simulink model "SiDynoReferenceApplication"  (R2020a)
settings: Solver=ode23tb  StartTime=0.0  StopTime=15000  RelTol=1e-3  EnableMultiTasking=on
model workspace (MAT data in the model file):
  DynOperatingPts : timeseries (value not decoded)
  MaxTurboSpd = 232000
  SteadyEngSpdCmdPts = [750 750 750 750 750 750 750 750 750 750 750 750 ... (225 elements, 15x15)]
  SteadyStateWaitLimit = 100
  SteadyTrqCmdPts = [15 30.3571428571 45.7142857143 61.0714285714 76.4285714286 91.7857142857 107.142857143 122.5 137.857142857 153.214285714 168.571428571 183.928571429 ... (225 elements, 15x15)]
undefined symbols (not defined in the file or in its folder): DynoResultsBlock, GenerateMappedEngineCalibrations, InjPw, RecalibrateSIController, ThrPosPctCmd, WgAreaPctCmd
libraries: autolibutils x2, simulink x2, autolibpowerinfoutils x1
(part 2 of 2)

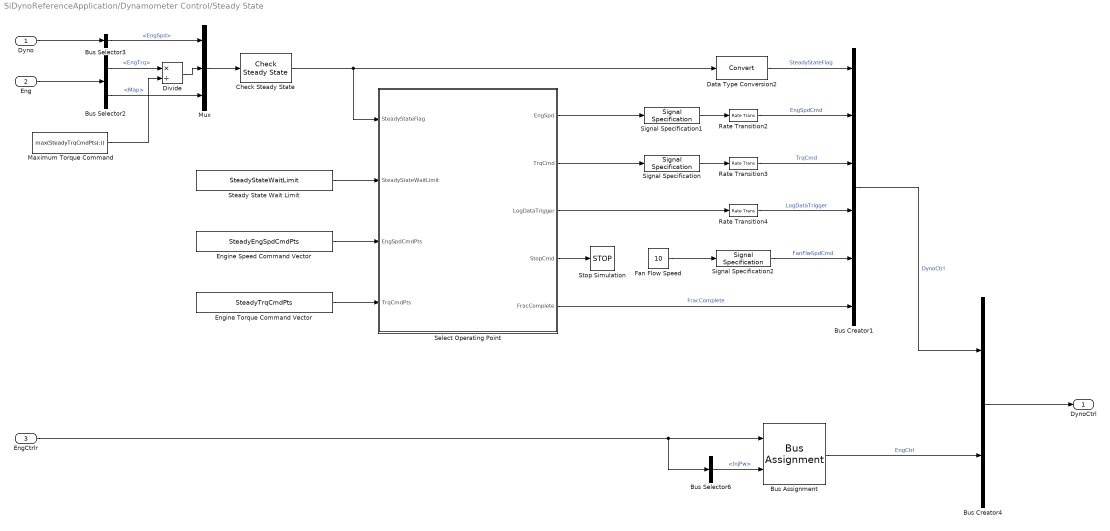
== system SiDynoReferenceApplication/Dynamometer Control/Steady State ==
  Dyno : Inport
  Eng : Inport  Port=2
  EngCtrlr : Inport  Port=3
  Bus Assignment : BusAssignment  AssignedSignals=InjPw
  Bus Creator1 : BusCreator  Inputs=6
  Bus Creator4 : BusCreator  Inputs=2
  Bus Selector2 : BusSelector  OutputSignals=EngPlnt.EngTrq,EngPlnt.Map
  Bus Selector3 : BusSelector  OutputSignals=DynoPlnt.EngSpd
  Bus Selector6 : BusSelector  OutputSignals=InjPw
  Check Steady State : autolibutils/Check Steady State  N=4  F=25  Ts=0.1  SteadyThresh=[0.25; 0.002; 2000]  HoldTime=1  aMode=aMode
      settings: SourceProductBaseCode=PW,MT,VE,VP
  Data Type Conversion2 : DataTypeConversion
  Divide : Product  Inputs=*/
  Engine Speed Command Vector : Constant  Value=SteadyEngSpdCmdPts
  Engine Torque Command Vector : Constant  Value=SteadyTrqCmdPts
  Fan Flow Speed : Constant  Value=10
  Maximum Torque Command : Constant  Value=max(SteadyTrqCmdPts(:))
  Mux : Mux  Inputs=3
  Rate Transition2 : RateTransition
  Rate Transition3 : RateTransition
  Rate Transition4 : RateTransition
  Select Operating Point : Stateflow chart  TreatAsAtomicUnit=on
  Signal Specification : SignalSpecification  Unit=N*m
  Signal Specification1 : SignalSpecification  Unit=rpm
  Signal Specification2 : SignalSpecification  Unit=m/s
  Steady State Wait Limit : Constant  Value=SteadyStateWaitLimit
  Stop Simulation : Stop
  DynoCtrl : Outport  VectorParamsAs1DForOutWhenUnconnected=off
  wires:
  Maximum Torque Command/1 -> Divide/2
  Divide/1 -> Mux/2
  Select Operating Point/5(FracComplete) -> Bus Creator1/6  "FracComplete"
  Signal Specification/1 -> Rate Transition3/1
  Signal Specification1/1 -> Rate Transition2/1
  Signal Specification2/1 -> Bus Creator1/5  "FanFlwSpdCmd"
  Fan Flow Speed/1 -> Signal Specification2/1
  Select Operating Point/4(StopCmd) -> Stop Simulation/1
  Engine Speed Command Vector/1 -> Select Operating Point/3(EngSpdCmdPts)
  Engine Torque Command Vector/1 -> Select Operating Point/4(TrqCmdPts)
  Select Operating Point/1(EngSpd) -> Signal Specification1/1
  Select Operating Point/2(TrqCmd) -> Signal Specification/1
  Select Operating Point/3(LogDataTrigger) -> Rate Transition4/1
  Rate Transition2/1 -> Bus Creator1/2  "EngSpdCmd"
  Rate Transition3/1 -> Bus Creator1/3  "TrqCmd"
  Rate Transition4/1 -> Bus Creator1/4  "LogDataTrigger"
  Data Type Conversion2/1 -> Bus Creator1/1  "SteadyStateFlag"
  Check Steady State/1 -> Select Operating Point/1(SteadyStateFlag), Data Type Conversion2/1
  Bus Creator4/1 -> DynoCtrl/1
  Bus Creator1/1 -> Bus Creator4/1  "DynoCtrl"
  Bus Assignment/1 -> Bus Creator4/2  "EngCtrl"
  Eng/1 -> Bus Selector2/1
  Dyno/1 -> Bus Selector3/1
  Mux/1 -> Check Steady State/1
  Bus Selector2/2 -> Mux/3  "<Map>"
  Bus Selector2/1 -> Divide/1  "<EngTrq>"
  Bus Selector3/1 -> Mux/1  "<EngSpd>"
  EngCtrlr/1 -> Bus Selector6/1, Bus Assignment/1
  Bus Selector6/1 -> Bus Assignment/2  "<InjPw>"
  Steady State Wait Limit/1 -> Select Operating Point/2(SteadyStateWaitLimit)

== system SiDynoReferenceApplication/Engine System/Dynamometer Engine Control ==
  Dyno : Inport
  Bus Selector : BusSelector  OutputSignals=DynoCtrl.EngCtrl
  Ctrl : Outport  VectorParamsAs1DForOutWhenUnconnected=off
  wires:
  Dyno/1 -> Bus Selector/1
  Bus Selector/1 -> Ctrl/1  "<EngCtrl>"

== system SiDynoReferenceApplication/Engine System/Engine Controller ==
  Env : Inport
  Dyno : Inport  Port=2
  EngPlnt : Inport  Port=3
  Engine Control Input : Subsystem
  Engine Control Output : Subsystem
  Engine Controller : ModelReference  ModelNameDialog=SiEngineController.slx  SimulationMode=Normal  OverrideUsingVariant=1  ModelReferenceVersion=1.306
  Mux : Mux  Inputs=3
  To Workspace : ToWorkspace  VariableName=Engine_Vars  SaveFormat=Timeseries  SampleTime=-1
  EngCtrlrOutput : Outport  VectorParamsAs1DForOutWhenUnconnected=off
  wires:
  Engine Controller/17 -> Engine Control Output/17(EstIntkPortFlw)
  Engine Controller/16 -> Engine Control Output/16(LoadCmd)
  Engine Controller/15 -> Engine Control Output/15(TrqCmdISC)
  Engine Controller/14 -> Engine Control Output/14(IntkSwirlVlvPosCmd)
  Engine Controller/13 -> Engine Control Output/13(ClsdLpFuelMult)
  Engine Controller/12 -> Engine Control Output/12(VarIntkRunLenCmd)
  Engine Controller/11 -> Engine Control Output/11(IntkVlvLiftCmd)
  Engine Controller/10 -> Engine Control Output/10(VarCompRatioPosCmd)
  Engine Controller/9 -> Engine Control Output/9(EgrVlvAreaPctCmd)
  Engine Controller/8 -> Engine Control Output/8(TurboRackPosCmd)
  Engine Controller/7 -> Engine Control Output/7(ExhCamPhaseCmd)
  Engine Controller/6 -> Engine Control Output/6(IntkCamPhaseCmd)
  Engine Controller/5 -> Engine Control Output/5(SpkAdv)
  Engine Controller/4 -> Engine Control Output/4(FuelMainSoi)
  Engine Controller/3 -> Engine Control Output/3(InjPw)
  Engine Controller/2 -> Engine Control Output/2(WgAreaPctCmd)
  Engine Controller/1 -> Engine Control Output/1(ThrPosPctCmd)
  Engine Control Input/17(AmbPrs) -> Engine Controller/17
  Engine Control Input/16(TurboSpd) -> Engine Controller/16
  Engine Control Input/15(IntkSwirlVlvPos) -> Engine Controller/15
  Engine Control Input/14(Afr) -> Mux/3, Engine Controller/14  "Air-Fuel"
  Engine Control Input/13(VarIntkRunLen) -> Engine Controller/13
  Engine Control Input/12(IntkVlvLift) -> Engine Controller/12
  Engine Control Input/11(VarCompRatioPos) -> Engine Controller/11
  Engine Control Input/10(EgrVlvAreaPct) -> Engine Controller/10
  Engine Control Input/9(TurboRackPos) -> Engine Controller/9
  Engine Control Input/8(ExhCamPhase) -> Engine Controller/8
  Engine Control Input/7(IntkCamPhase) -> Engine Controller/7
  Engine Control Input/6(WgAreaPct) -> Engine Controller/6
  Engine Control Input/5(ThrPosPct) -> Engine Controller/5
  Engine Control Input/4(Mat) -> Engine Controller/4
  Engine Control Input/3(Map) -> Engine Controller/3, Mux/2  "MAP"
  Engine Control Input/2(EngSpd) -> Engine Controller/2, Mux/1  "EngineSpeed"
  Engine Control Input/1(TrqCmd) -> Engine Controller/1
  Engine Control Output/1(EngCtrlrOutput) -> EngCtrlrOutput/1
  Dyno/1 -> Engine Control Input/1(Dyno)
  Env/1 -> Engine Control Input/2(Env)
  EngPlnt/1 -> Engine Control Input/3(VehPlnt)
  Engine Control Input/18(IgSw) -> Engine Controller/18
  Engine Control Input/19(Iat) -> Engine Controller/19
  Engine Control Input/20(Ect) -> Engine Controller/20
  Engine Control Input/21(EgrVlvDeltaPrs) -> Engine Controller/21
  Engine Control Input/22(EgrVlvInTemp) -> Engine Controller/22
  Mux/1 -> To Workspace/1

== system SiDynoReferenceApplication/Engine System/Engine Plant ==
  Env : Inport
  Ctrl : Inport  Port=2
  Dyno : Inport  Port=3
  Engine : Subsystem  Variant=on  VariantControlMode=Label  LabelModeActiveChoice=SiEngine
      mask init:
      | GenerateMappedEngineCalibrations(gcb, 'UpdateParentIcon');
  Engine Plant Input : Subsystem
  Engine Plant Output : Subsystem
  EngPlnt : Outport  VectorParamsAs1DForOutWhenUnconnected=off
  wires:
  Engine/14(IntkSwirlVlvPos) -> Engine Plant Output/14(IntkSwirlVlvPos)
  Engine/13(VarIntkRunLen) -> Engine Plant Output/13(VarIntkRunLen)
  Engine/12(IntkVlvLift) -> Engine Plant Output/12(IntkVlvLift)
  Engine/11(VarCompRatioPos) -> Engine Plant Output/11(VarCompRatioPos)
  Engine Plant Input/19(UndHdFlwVel) -> Engine/19(UndHdFlwVel)
  Engine Plant Input/18(EngSpd) -> Engine/18(EngSpd)
  Engine Plant Input/17(AmbPrs) -> Engine/17(AmbPrs)
  Engine Plant Input/16(AmbTemp) -> Engine/16(AmbTemp)
  Engine Plant Input/15(TrqCmd) -> Engine/15(TrqCmd)
  Engine Plant Input/14(IntkSwirlVlvPosCmd) -> Engine/14(IntkSwirlVlvPosCmd)
  Engine Plant Input/13(ClsdLpFuelMult) -> Engine/13(ClsdLpFuelMult)
  Engine Plant Input/12(VarIntkRunLenCmd) -> Engine/12(VarIntkRunLenCmd)
  Engine Plant Input/11(IntkVlvLiftCmd) -> Engine/11(IntkVlvLiftCmd)
  Engine Plant Input/10(VarCompRatioPosCmd) -> Engine/10(VarCompRatioPosCmd)
  Engine Plant Input/9(EgrVlvAreaPctCmd) -> Engine/9(EgrVlvAreaPctCmd)
  Engine Plant Input/1(ThrPosPctCmd) -> Engine/1(ThrPosPctCmd)
  Engine Plant Input/8(TurboRackPosCmd) -> Engine/8(TurboRackPosCmd)
  Engine Plant Input/2(WgAreaPctCmd) -> Engine/2(WgAreaPctCmd)
  Engine Plant Input/7(ExhCamPhaseCmd) -> Engine/7(ExhCamPhaseCmd)
  Engine Plant Input/3(InjPw) -> Engine/3(InjPw)
  Engine Plant Input/6(IntkCamPhaseCmd) -> Engine/6(IntkCamPhaseCmd)
  Engine Plant Input/4(FuelMainSoi) -> Engine/4(FuelMainSoi)
  Engine Plant Input/5(SpkAdv) -> Engine/5(SpkAdv)
  Engine/34(TP CO2) -> Engine Plant Output/34(TP CO2)
  Engine/33(TP NOx) -> Engine Plant Output/33(TP NOx)
  Engine/32(TP CO) -> Engine Plant Output/32(TP CO)
  Engine/31(TP HC) -> Engine Plant Output/31(TP HC)
  Engine/30(BSFC) -> Engine Plant Output/30(BSFC)
  Engine/29(IntercoolerTempOut) -> Engine Plant Output/29(IntercoolerTempOut)
  Engine/28(EgrCoolerTempOut) -> Engine Plant Output/28(EgrCoolerTempOut)
  Engine/27(EgrMassFlwRate) -> Engine Plant Output/27(EgrMassFlwRate)
  Engine/26(EgrPct) -> Engine Plant Output/26(EgrPct)
  Engine/25(CompTempOut) -> Engine Plant Output/25(CompTempOut)
  Engine/24(TurbTempOut) -> Engine Plant Output/24(TurbTempOut)
  Engine/23(CompPrsRatio) -> Engine Plant Output/23(CompPrsRatio)
  Engine/22(TurbPrsRatio) -> Engine Plant Output/22(TurbPrsRatio)
  Engine/21(TurboSpd) -> Engine Plant Output/21(TurboSpd)
  Engine/20(Afr) -> Engine Plant Output/20(Afr)
  Engine/19(ExhManGasTemp) -> Engine Plant Output/19(ExhManGasTemp)
  Engine/18(NormAirChrg) -> Engine Plant Output/18(NormAirChrg)
  Engine/17(IntkPortFlw) -> Engine Plant Output/17(IntkPortFlow)
  Engine/15(FuelFlw) -> Engine Plant Output/15(FuelFlw)
  Engine/10(EgrVlvAreaPct) -> Engine Plant Output/10(EgrVlvAreaPct)
  Engine/9(TurboRackPos) -> Engine Plant Output/9(TurboRackPos)
  Engine/8(ExhCamPhase) -> Engine Plant Output/8(ExhCamPhase)
  Engine/7(IntkCamPhase) -> Engine Plant Output/7(IntkCamPhase)
  Engine/6(WgAreaPct) -> Engine Plant Output/6(WgAreaPct)
  Engine/5(ThrPosPct) -> Engine Plant Output/5(ThrPosPct)
  Engine/4(Mat) -> Engine Plant Output/4(Mat)
  Engine/3(Map) -> Engine Plant Output/3(Map)
  Engine/2(EngSpdOut) -> Engine Plant Output/2(EngSpd)
  Engine/1(EngTrq) -> Engine Plant Output/1(EngTrq)
  Dyno/1 -> Engine Plant Input/3(Dyno)
  Engine Plant Output/1(EngFdbkOut) -> EngPlnt/1
  Ctrl/1 -> Engine Plant Input/1(Ctrl)
  Env/1 -> Engine Plant Input/2(Env)
  Engine/36(Ect) -> Engine Plant Output/36(Ect)
  Engine/37(EgrVlvDeltaPrs) -> Engine Plant Output/37(EgrVlvDeltaPrs)
  Engine/38(EgrVlvInTemp) -> Engine Plant Output/38(EgrVlvInTemp)
  Engine/35(Iat) -> Engine Plant Output/35(Iat)
  Engine/16(FuelVolFlw) -> Engine Plant Output/16(FuelVolFlw)

== system SiDynoReferenceApplication/Performance Monitor/Dynamic Logging ==
  LogData : Inport
  Bus Creator : BusCreator  Inputs=9
  Bus Selector : BusSelector  OutputSignals=Torque command (N*m),Measured engine torque (N*m),Engine speed (rpm),BSFC (g/(kW*hr)),Fuel mass flow rate (g/s),Intake port mass flow rate (g/s),Turbocharger shaft speed (rpm),Intake manifold pressure (kPa),Time (s)
  To Workspace : ToWorkspace  VariableName=DynamicDynoSimOut  SampleTime=-1
      settings: Decimation=100
  wires:
  Bus Selector/7 -> Bus Creator/7  "<Turbocharger shaft speed (rpm)>"
  Bus Selector/1 -> Bus Creator/1  "<Torque command (N*m)>"
  Bus Selector/6 -> Bus Creator/6  "<Intake port mass flow rate (g/s)>"
  Bus Selector/4 -> Bus Creator/4  "<BSFC (g/(kW*hr))>"
  Bus Selector/5 -> Bus Creator/5  "<Fuel mass flow rate (g/s)>"
  Bus Selector/3 -> Bus Creator/3  "<Engine speed (rpm)>"
  Bus Selector/2 -> Bus Creator/2  "<Measured engine torque (N*m)>"
  Bus Selector/8 -> Bus Creator/8  "<Intake manifold pressure (kPa)>"
  Bus Selector/9 -> Bus Creator/9  "<Time (s)>"
  Bus Creator/1 -> To Workspace/1
  LogData/1 -> Bus Selector/1

== system SiDynoReferenceApplication/Performance Monitor/Steady State Logging ==
  LogData : Inport
  Trigger : TriggerPort  VariantControl=Variant  PortDimensions=1
  To Workspace : ToWorkspace  VariableName=SteadyDynoSimOut  SampleTime=-1
  wires:
  LogData/1 -> To Workspace/1

== system SiDynoReferenceApplication/Performance Monitor/Waitbar ==
  FracComplete : Inport
  Function-Call Generator : simulink/Ports & Subsystems/Function-Call Generator  sample_time=5  numberOfIterations=1
  Function-Call Subsystem : Subsystem  TreatAsAtomicUnit=on
  Rate Transition : RateTransition
  wires:
  Rate Transition/1 -> Function-Call Subsystem/1(FracComplete)
  Function-Call Generator/1 -> Function-Call Subsystem/Trigger
  FracComplete/1 -> Rate Transition/1

== system SiDynoReferenceApplication/Dynamometer/Dynamometer Plant/Cooling Fan ==
  FanFlwSpdCmd : Inport
  Bus Selector : BusSelector  OutputSignals=FanFlwSpdCmd
  Cooling Fan Dynamics : TransferFcn  Denominator=[0.4 1]
  FanFlwSpd : Outport  VectorParamsAs1DForOutWhenUnconnected=off
  wires:
  FanFlwSpdCmd/1 -> Bus Selector/1
  Cooling Fan Dynamics/1 -> FanFlwSpd/1
  Bus Selector/1 -> Cooling Fan Dynamics/1  "<FanFlwSpdCmd>"

== system SiDynoReferenceApplication/Dynamometer/Dynamometer Plant/Dynamometer Load Motor ==
  DynoCtrl : Inport
  Bus Selector : BusSelector  OutputSignals=EngSpdCmd
  Dyno Dynamics : TransferFcn  Denominator=[0.1 1]
  EngSpd : Outport  VectorParamsAs1DForOutWhenUnconnected=off
  wires:
  Dyno Dynamics/1 -> EngSpd/1
  DynoCtrl/1 -> Bus Selector/1
  Bus Selector/1 -> Dyno Dynamics/1  "<EngSpdCmd>"

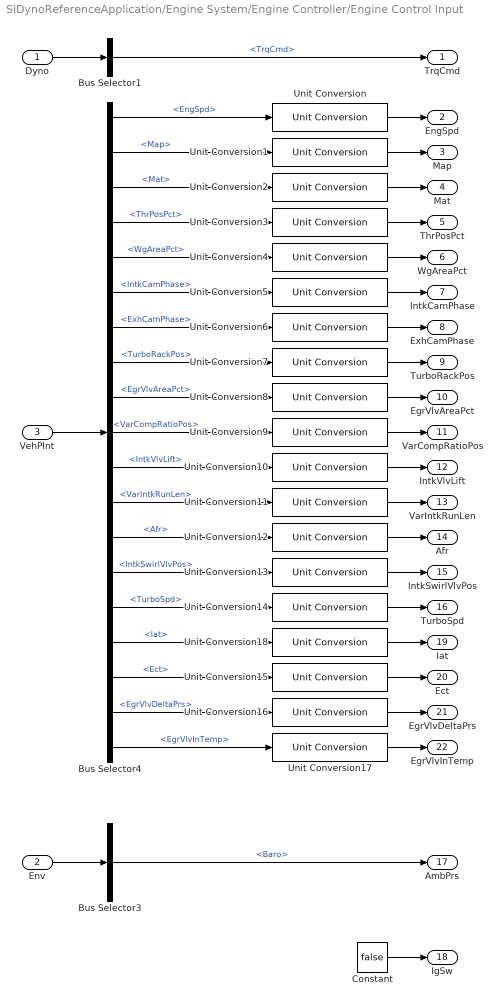
== system SiDynoReferenceApplication/Engine System/Engine Controller/Engine Control Input ==
  Dyno : Inport
  Env : Inport  Port=2
  VehPlnt : Inport  Port=3
  Bus Selector1 : BusSelector  OutputSignals=DynoCtrl.TrqCmd
  Bus Selector3 : BusSelector  OutputSignals=Baro
  Bus Selector4 : BusSelector  OutputSignals=EngSpd,Map,Mat,ThrPosPct,WgAreaPct,IntkCamPhase,ExhCamPhase,TurboRackPos,EgrVlvAreaPct,VarCompRatioPos,IntkVlvLift,VarIntkRunLen,Afr,IntkSwirlVlvPos,TurboSpd,Iat,Ect,EgrVlvDeltaPrs,EgrVlvInTemp
  Constant : Constant  Value=false
  Unit Conversion{,1..18} (19 alike) : UnitConversion
  TrqCmd : Outport  VectorParamsAs1DForOutWhenUnconnected=off
  EngSpd : Outport  Port=2  VectorParamsAs1DForOutWhenUnconnected=off
  Map : Outport  Port=3  VectorParamsAs1DForOutWhenUnconnected=off
  Mat : Outport  Port=4  VectorParamsAs1DForOutWhenUnconnected=off
  ThrPosPct : Outport  Port=5  VectorParamsAs1DForOutWhenUnconnected=off
  WgAreaPct : Outport  Port=6  VectorParamsAs1DForOutWhenUnconnected=off
  IntkCamPhase : Outport  Port=7  VectorParamsAs1DForOutWhenUnconnected=off
  ExhCamPhase : Outport  Port=8  VectorParamsAs1DForOutWhenUnconnected=off
  TurboRackPos : Outport  Port=9  VectorParamsAs1DForOutWhenUnconnected=off
  EgrVlvAreaPct : Outport  Port=10  VectorParamsAs1DForOutWhenUnconnected=off
  VarCompRatioPos : Outport  Port=11  VectorParamsAs1DForOutWhenUnconnected=off
  IntkVlvLift : Outport  Port=12  VectorParamsAs1DForOutWhenUnconnected=off
  VarIntkRunLen : Outport  Port=13  VectorParamsAs1DForOutWhenUnconnected=off
  Afr : Outport  Port=14  VectorParamsAs1DForOutWhenUnconnected=off
  IntkSwirlVlvPos : Outport  Port=15  VectorParamsAs1DForOutWhenUnconnected=off
  TurboSpd : Outport  Port=16  VectorParamsAs1DForOutWhenUnconnected=off
  AmbPrs : Outport  Port=17  VectorParamsAs1DForOutWhenUnconnected=off
  IgSw : Outport  Port=18  VectorParamsAs1DForOutWhenUnconnected=off
  Iat : Outport  Port=19  VectorParamsAs1DForOutWhenUnconnected=off
  Ect : Outport  Port=20  VectorParamsAs1DForOutWhenUnconnected=off
  EgrVlvDeltaPrs : Outport  Port=21  VectorParamsAs1DForOutWhenUnconnected=off
  EgrVlvInTemp : Outport  Port=22  VectorParamsAs1DForOutWhenUnconnected=off
  wires:
  Unit Conversion14/1 -> TurboSpd/1
  Unit Conversion13/1 -> IntkSwirlVlvPos/1
  Unit Conversion12/1 -> Afr/1
  Unit Conversion11/1 -> VarIntkRunLen/1
  Unit Conversion8/1 -> EgrVlvAreaPct/1
  Unit Conversion9/1 -> VarCompRatioPos/1
  Unit Conversion10/1 -> IntkVlvLift/1
  Unit Conversion7/1 -> TurboRackPos/1
  Unit Conversion5/1 -> IntkCamPhase/1
  Unit Conversion6/1 -> ExhCamPhase/1
  Unit Conversion4/1 -> WgAreaPct/1
  Unit Conversion3/1 -> ThrPosPct/1
  Unit Conversion2/1 -> Mat/1
  Unit Conversion1/1 -> Map/1
  Unit Conversion/1 -> EngSpd/1
  Dyno/1 -> Bus Selector1/1
  Env/1 -> Bus Selector3/1
  VehPlnt/1 -> Bus Selector4/1
  Constant/1 -> IgSw/1
  Unit Conversion15/1 -> Ect/1
  Unit Conversion17/1 -> EgrVlvInTemp/1
  Unit Conversion16/1 -> EgrVlvDeltaPrs/1
  Unit Conversion18/1 -> Iat/1
  Bus Selector1/1 -> TrqCmd/1  "<TrqCmd>"
  Bus Selector4/1 -> Unit Conversion/1  "<EngSpd>"
  Bus Selector4/2 -> Unit Conversion1/1  "<Map>"
  Bus Selector4/3 -> Unit Conversion2/1  "<Mat>"
  Bus Selector4/4 -> Unit Conversion3/1  "<ThrPosPct>"
  Bus Selector4/5 -> Unit Conversion4/1  "<WgAreaPct>"
  Bus Selector4/6 -> Unit Conversion5/1  "<IntkCamPhase>"
  Bus Selector4/7 -> Unit Conversion6/1  "<ExhCamPhase>"
  Bus Selector4/8 -> Unit Conversion7/1  "<TurboRackPos>"
  Bus Selector4/9 -> Unit Conversion8/1  "<EgrVlvAreaPct>"
  Bus Selector4/10 -> Unit Conversion9/1  "<VarCompRatioPos>"
  Bus Selector4/11 -> Unit Conversion10/1  "<IntkVlvLift>"
  Bus Selector4/12 -> Unit Conversion11/1  "<VarIntkRunLen>"
  Bus Selector4/13 -> Unit Conversion12/1  "<Afr>"
  Bus Selector4/14 -> Unit Conversion13/1  "<IntkSwirlVlvPos>"
  Bus Selector4/15 -> Unit Conversion14/1  "<TurboSpd>"
  Bus Selector4/16 -> Unit Conversion18/1  "<Iat>"
  Bus Selector4/17 -> Unit Conversion15/1  "<Ect>"
  Bus Selector4/18 -> Unit Conversion16/1  "<EgrVlvDeltaPrs>"
  Bus Selector4/19 -> Unit Conversion17/1  "<EgrVlvInTemp>"
  Bus Selector3/1 -> AmbPrs/1  "<Baro>"

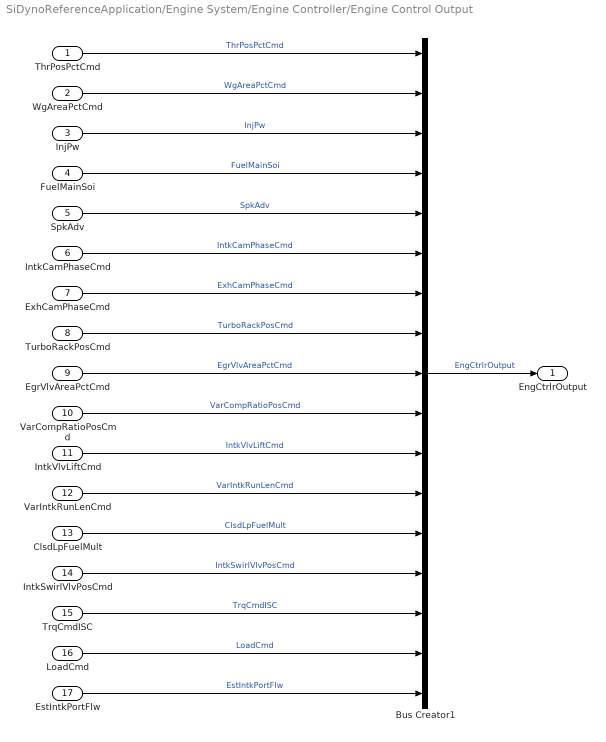
== system SiDynoReferenceApplication/Engine System/Engine Controller/Engine Control Output ==
  ThrPosPctCmd : Inport
  WgAreaPctCmd : Inport  Port=2
  InjPw : Inport  Port=3
  FuelMainSoi : Inport  Port=4
  SpkAdv : Inport  Port=5
  IntkCamPhaseCmd : Inport  Port=6
  ExhCamPhaseCmd : Inport  Port=7
  TurboRackPosCmd : Inport  Port=8
  EgrVlvAreaPctCmd : Inport  Port=9
  VarCompRatioPosCmd : Inport  Port=10
  IntkVlvLiftCmd : Inport  Port=11
  VarIntkRunLenCmd : Inport  Port=12
  ClsdLpFuelMult : Inport  Port=13
  IntkSwirlVlvPosCmd : Inport  Port=14
  TrqCmdISC : Inport  Port=15
  LoadCmd : Inport  Port=16
  EstIntkPortFlw : Inport  Port=17
  Bus Creator1 : BusCreator  Inputs=17
  EngCtrlrOutput : Outport  VectorParamsAs1DForOutWhenUnconnected=off
  wires:
  VarCompRatioPosCmd/1 -> Bus Creator1/10  "VarCompRatioPosCmd"
  IntkSwirlVlvPosCmd/1 -> Bus Creator1/14  "IntkSwirlVlvPosCmd"
  IntkVlvLiftCmd/1 -> Bus Creator1/11  "IntkVlvLiftCmd"
  VarIntkRunLenCmd/1 -> Bus Creator1/12  "VarIntkRunLenCmd"
  ClsdLpFuelMult/1 -> Bus Creator1/13  "ClsdLpFuelMult"
  TurboRackPosCmd/1 -> Bus Creator1/8  "TurboRackPosCmd"
  TrqCmdISC/1 -> Bus Creator1/15  "TrqCmdISC"
  ExhCamPhaseCmd/1 -> Bus Creator1/7  "ExhCamPhaseCmd"
  IntkCamPhaseCmd/1 -> Bus Creator1/6  "IntkCamPhaseCmd"
  InjPw/1 -> Bus Creator1/3  "InjPw"
  WgAreaPctCmd/1 -> Bus Creator1/2  "WgAreaPctCmd"
  Bus Creator1/1 -> EngCtrlrOutput/1  "EngCtrlrOutput"
  EgrVlvAreaPctCmd/1 -> Bus Creator1/9  "EgrVlvAreaPctCmd"
  LoadCmd/1 -> Bus Creator1/16  "LoadCmd"
  ThrPosPctCmd/1 -> Bus Creator1/1  "ThrPosPctCmd"
  FuelMainSoi/1 -> Bus Creator1/4  "FuelMainSoi"
  SpkAdv/1 -> Bus Creator1/5  "SpkAdv"
  EstIntkPortFlw/1 -> Bus Creator1/17  "EstIntkPortFlw"

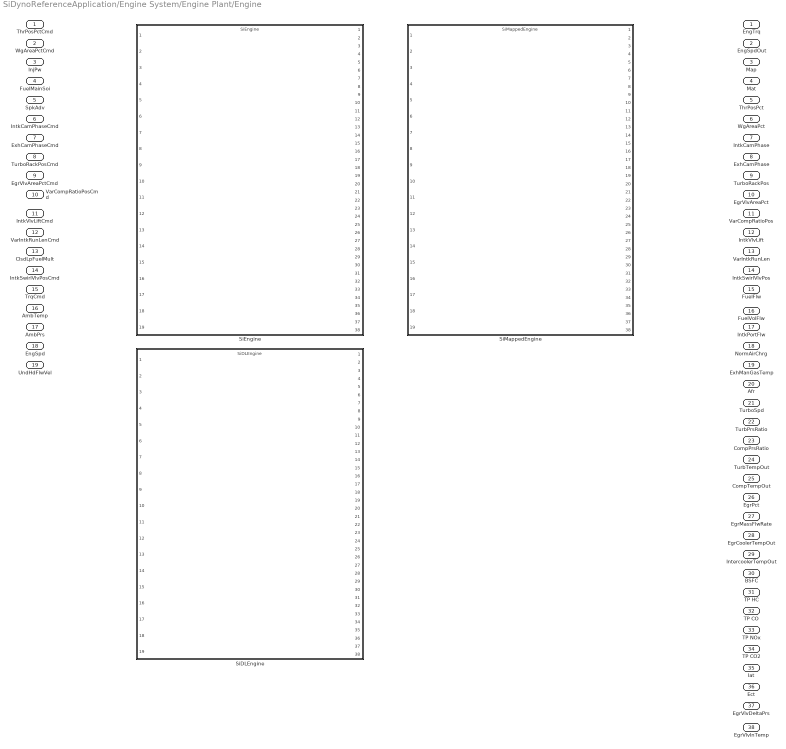
== system SiDynoReferenceApplication/Engine System/Engine Plant/Engine ==
  ThrPosPctCmd : Inport
  WgAreaPctCmd : Inport  Port=2
  InjPw : Inport  Port=3
  FuelMainSoi : Inport  Port=4
  SpkAdv : Inport  Port=5
  IntkCamPhaseCmd : Inport  Port=6
  ExhCamPhaseCmd : Inport  Port=7
  TurboRackPosCmd : Inport  Port=8
  EgrVlvAreaPctCmd : Inport  Port=9
  VarCompRatioPosCmd : Inport  Port=10
  IntkVlvLiftCmd : Inport  Port=11
  VarIntkRunLenCmd : Inport  Port=12
  ClsdLpFuelMult : Inport  Port=13
  IntkSwirlVlvPosCmd : Inport  Port=14
  TrqCmd : Inport  Port=15
  AmbTemp : Inport  Port=16
  AmbPrs : Inport  Port=17
  EngSpd : Inport  Port=18
  UndHdFlwVel : Inport  Port=19
  SiDLEngine : ModelReference  ModelNameDialog=SiDLEngine  SimulationMode=Normal  VariantControl=SiDLEngine  ModelReferenceVersion=1.459
  SiEngine : ModelReference  ModelNameDialog=SiEngine.slx  SimulationMode=Normal  VariantControl=SiEngine  ModelReferenceVersion=1.573
  SiMappedEngine : ModelReference  ModelNameDialog=SiMappedEngine.slx  SimulationMode=Normal  VariantControl=SiMappedEngine  ModelReferenceVersion=1.331
  EngTrq : Outport  VectorParamsAs1DForOutWhenUnconnected=off
  EngSpdOut : Outport  Port=2  VectorParamsAs1DForOutWhenUnconnected=off
  Map : Outport  Port=3  VectorParamsAs1DForOutWhenUnconnected=off
  Mat : Outport  Port=4  VectorParamsAs1DForOutWhenUnconnected=off
  ThrPosPct : Outport  Port=5  VectorParamsAs1DForOutWhenUnconnected=off
  WgAreaPct : Outport  Port=6  VectorParamsAs1DForOutWhenUnconnected=off
  IntkCamPhase : Outport  Port=7  VectorParamsAs1DForOutWhenUnconnected=off
  ExhCamPhase : Outport  Port=8  VectorParamsAs1DForOutWhenUnconnected=off
  TurboRackPos : Outport  Port=9  VectorParamsAs1DForOutWhenUnconnected=off
  EgrVlvAreaPct : Outport  Port=10  VectorParamsAs1DForOutWhenUnconnected=off
  VarCompRatioPos : Outport  Port=11  VectorParamsAs1DForOutWhenUnconnected=off
  IntkVlvLift : Outport  Port=12  VectorParamsAs1DForOutWhenUnconnected=off
  VarIntkRunLen : Outport  Port=13  VectorParamsAs1DForOutWhenUnconnected=off
  IntkSwirlVlvPos : Outport  Port=14  VectorParamsAs1DForOutWhenUnconnected=off
  FuelFlw : Outport  Port=15  VectorParamsAs1DForOutWhenUnconnected=off
  FuelVolFlw : Outport  Port=16  VectorParamsAs1DForOutWhenUnconnected=off
  IntkPortFlw : Outport  Port=17  VectorParamsAs1DForOutWhenUnconnected=off
  NormAirChrg : Outport  Port=18  VectorParamsAs1DForOutWhenUnconnected=off
  ExhManGasTemp : Outport  Port=19  VectorParamsAs1DForOutWhenUnconnected=off
  Afr : Outport  Port=20  VectorParamsAs1DForOutWhenUnconnected=off
  TurboSpd : Outport  Port=21  VectorParamsAs1DForOutWhenUnconnected=off
  TurbPrsRatio : Outport  Port=22  VectorParamsAs1DForOutWhenUnconnected=off
  CompPrsRatio : Outport  Port=23  VectorParamsAs1DForOutWhenUnconnected=off
  TurbTempOut : Outport  Port=24  VectorParamsAs1DForOutWhenUnconnected=off
  CompTempOut : Outport  Port=25  VectorParamsAs1DForOutWhenUnconnected=off
  EgrPct : Outport  Port=26  VectorParamsAs1DForOutWhenUnconnected=off
  EgrMassFlwRate : Outport  Port=27  VectorParamsAs1DForOutWhenUnconnected=off
  EgrCoolerTempOut : Outport  Port=28  VectorParamsAs1DForOutWhenUnconnected=off
  IntercoolerTempOut : Outport  Port=29  VectorParamsAs1DForOutWhenUnconnected=off
  BSFC : Outport  Port=30  VectorParamsAs1DForOutWhenUnconnected=off
  TP HC : Outport  Port=31  VectorParamsAs1DForOutWhenUnconnected=off
  TP CO : Outport  Port=32  VectorParamsAs1DForOutWhenUnconnected=off
  TP NOx : Outport  Port=33  VectorParamsAs1DForOutWhenUnconnected=off
  TP CO2 : Outport  Port=34  VectorParamsAs1DForOutWhenUnconnected=off
  Iat : Outport  Port=35  VectorParamsAs1DForOutWhenUnconnected=off
  Ect : Outport  Port=36  VectorParamsAs1DForOutWhenUnconnected=off
  EgrVlvDeltaPrs : Outport  Port=37  VectorParamsAs1DForOutWhenUnconnected=off
  EgrVlvInTemp : Outport  Port=38  VectorParamsAs1DForOutWhenUnconnected=off

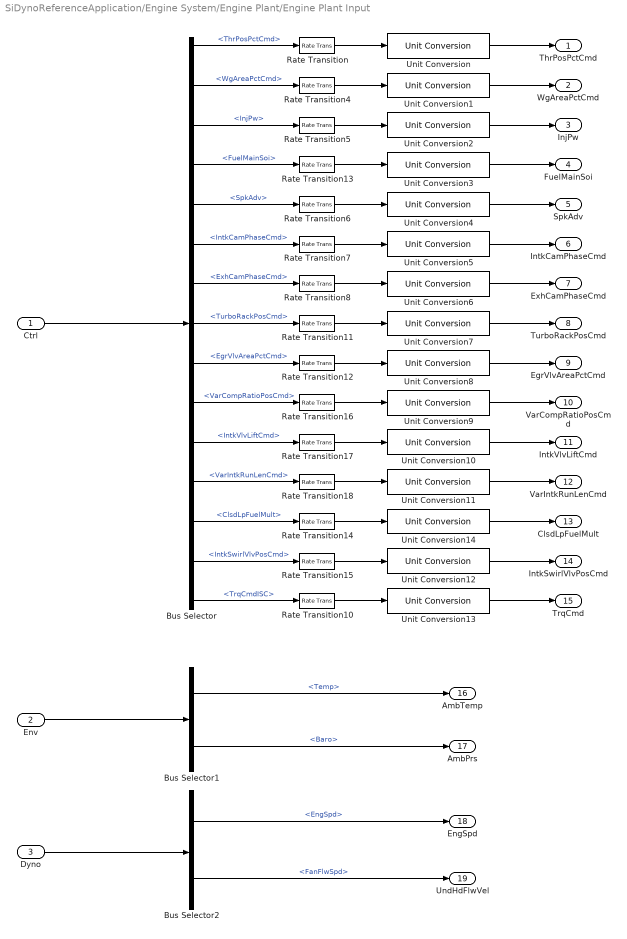
== system SiDynoReferenceApplication/Engine System/Engine Plant/Engine Plant Input ==
  Ctrl : Inport
  Env : Inport  Port=2
  Dyno : Inport  Port=3
  Bus Selector : BusSelector  OutputSignals=ThrPosPctCmd,WgAreaPctCmd,InjPw,FuelMainSoi,SpkAdv,IntkCamPhaseCmd,ExhCamPhaseCmd,TurboRackPosCmd,EgrVlvAreaPctCmd,VarCompRatioPosCmd,IntkVlvLiftCmd,VarIntkRunLenCmd,ClsdLpFuelMult,IntkSwirlVlvPosCmd,TrqCmdISC
  Bus Selector1 : BusSelector  OutputSignals=Temp,Baro
  Bus Selector2 : BusSelector  OutputSignals=DynoPlnt.EngSpd,DynoPlnt.FanFlwSpd
  Rate Transition{,4..8,10..18} (15 alike) : RateTransition  Deterministic=off
  Unit Conversion{,1..14} (15 alike) : UnitConversion
  ThrPosPctCmd : Outport  VectorParamsAs1DForOutWhenUnconnected=off
  WgAreaPctCmd : Outport  Port=2  VectorParamsAs1DForOutWhenUnconnected=off
  InjPw : Outport  Port=3  VectorParamsAs1DForOutWhenUnconnected=off
  FuelMainSoi : Outport  Port=4  VectorParamsAs1DForOutWhenUnconnected=off
  SpkAdv : Outport  Port=5  VectorParamsAs1DForOutWhenUnconnected=off
  IntkCamPhaseCmd : Outport  Port=6  VectorParamsAs1DForOutWhenUnconnected=off
  ExhCamPhaseCmd : Outport  Port=7  VectorParamsAs1DForOutWhenUnconnected=off
  TurboRackPosCmd : Outport  Port=8  VectorParamsAs1DForOutWhenUnconnected=off
  EgrVlvAreaPctCmd : Outport  Port=9  VectorParamsAs1DForOutWhenUnconnected=off
  VarCompRatioPosCmd : Outport  Port=10  VectorParamsAs1DForOutWhenUnconnected=off
  IntkVlvLiftCmd : Outport  Port=11  VectorParamsAs1DForOutWhenUnconnected=off
  VarIntkRunLenCmd : Outport  Port=12  VectorParamsAs1DForOutWhenUnconnected=off
  ClsdLpFuelMult : Outport  Port=13  VectorParamsAs1DForOutWhenUnconnected=off
  IntkSwirlVlvPosCmd : Outport  Port=14  VectorParamsAs1DForOutWhenUnconnected=off
  TrqCmd : Outport  Port=15  VectorParamsAs1DForOutWhenUnconnected=off
  AmbTemp : Outport  Port=16  VectorParamsAs1DForOutWhenUnconnected=off
  AmbPrs : Outport  Port=17  VectorParamsAs1DForOutWhenUnconnected=off
  EngSpd : Outport  Port=18  VectorParamsAs1DForOutWhenUnconnected=off
  UndHdFlwVel : Outport  Port=19  VectorParamsAs1DForOutWhenUnconnected=off
  wires:
  Unit Conversion12/1 -> IntkSwirlVlvPosCmd/1
  Unit Conversion14/1 -> ClsdLpFuelMult/1
  Unit Conversion13/1 -> TrqCmd/1
  Unit Conversion9/1 -> VarCompRatioPosCmd/1
  Unit Conversion11/1 -> VarIntkRunLenCmd/1
  Unit Conversion10/1 -> IntkVlvLiftCmd/1
  Unit Conversion7/1 -> TurboRackPosCmd/1
  Unit Conversion6/1 -> ExhCamPhaseCmd/1
  Unit Conversion8/1 -> EgrVlvAreaPctCmd/1
  Unit Conversion5/1 -> IntkCamPhaseCmd/1
  Unit Conversion4/1 -> SpkAdv/1
  Unit Conversion3/1 -> FuelMainSoi/1
  Unit Conversion2/1 -> InjPw/1
  Unit Conversion1/1 -> WgAreaPctCmd/1
  Unit Conversion/1 -> ThrPosPctCmd/1
  Ctrl/1 -> Bus Selector/1
  Bus Selector/14 -> Rate Transition15/1  "<IntkSwirlVlvPosCmd>"
  Bus Selector/13 -> Rate Transition14/1  "<ClsdLpFuelMult>"
  Rate Transition15/1 -> Unit Conversion12/1
  Rate Transition14/1 -> Unit Conversion14/1
  Bus Selector/12 -> Rate Transition18/1  "<VarIntkRunLenCmd>"
  Rate Transition18/1 -> Unit Conversion11/1
  Bus Selector/11 -> Rate Transition17/1  "<IntkVlvLiftCmd>"
  Rate Transition17/1 -> Unit Conversion10/1
  Bus Selector/10 -> Rate Transition16/1  "<VarCompRatioPosCmd>"
  Rate Transition16/1 -> Unit Conversion9/1
  Rate Transition13/1 -> Unit Conversion3/1
  Bus Selector2/2 -> UndHdFlwVel/1  "<FanFlwSpd>"
  Bus Selector/1 -> Rate Transition/1  "<ThrPosPctCmd>"
  Rate Transition/1 -> Unit Conversion/1
  Env/1 -> Bus Selector1/1
  Bus Selector1/2 -> AmbPrs/1  "<Baro>"
  Dyno/1 -> Bus Selector2/1
  Bus Selector2/1 -> EngSpd/1  "<EngSpd>"
  Bus Selector1/1 -> AmbTemp/1  "<Temp>"
  Rate Transition4/1 -> Unit Conversion1/1
  Bus Selector/2 -> Rate Transition4/1  "<WgAreaPctCmd>"
  Rate Transition5/1 -> Unit Conversion2/1
  Bus Selector/3 -> Rate Transition5/1  "<InjPw>"
  Rate Transition6/1 -> Unit Conversion4/1
  Bus Selector/5 -> Rate Transition6/1  "<SpkAdv>"
  Rate Transition7/1 -> Unit Conversion5/1
  Bus Selector/6 -> Rate Transition7/1  "<IntkCamPhaseCmd>"
  Rate Transition8/1 -> Unit Conversion6/1
  Bus Selector/7 -> Rate Transition8/1  "<ExhCamPhaseCmd>"
  Rate Transition10/1 -> Unit Conversion13/1
  Bus Selector/15 -> Rate Transition10/1  "<TrqCmdISC>"
  Rate Transition11/1 -> Unit Conversion7/1
  Rate Transition12/1 -> Unit Conversion8/1
  Bus Selector/8 -> Rate Transition11/1  "<TurboRackPosCmd>"
  Bus Selector/9 -> Rate Transition12/1  "<EgrVlvAreaPctCmd>"
  Bus Selector/4 -> Rate Transition13/1  "<FuelMainSoi>"

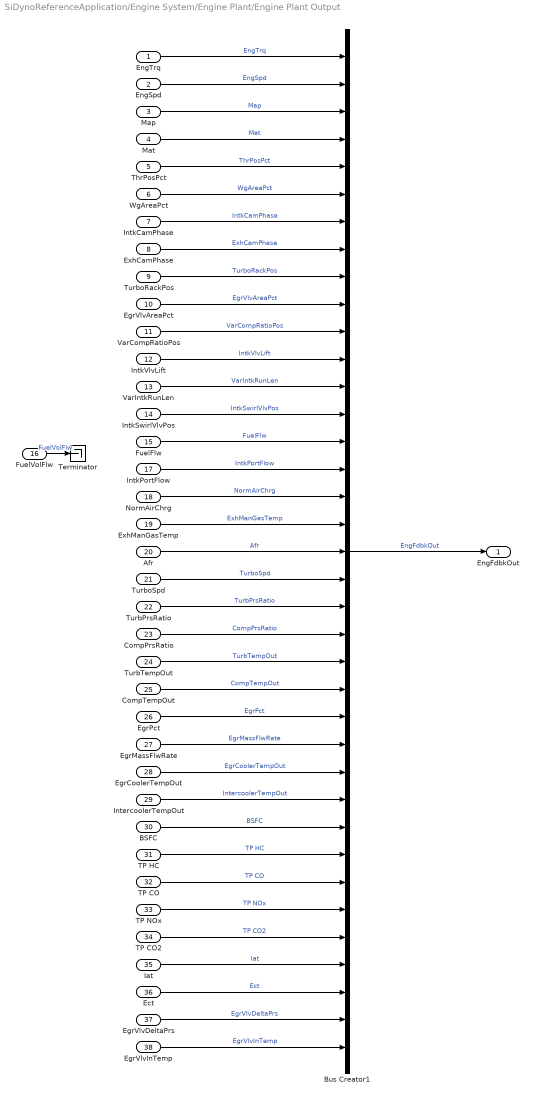
== system SiDynoReferenceApplication/Engine System/Engine Plant/Engine Plant Output ==
  EngTrq : Inport
  EngSpd : Inport  Port=2
  Map : Inport  Port=3
  Mat : Inport  Port=4
  ThrPosPct : Inport  Port=5
  WgAreaPct : Inport  Port=6
  IntkCamPhase : Inport  Port=7
  ExhCamPhase : Inport  Port=8
  TurboRackPos : Inport  Port=9
  EgrVlvAreaPct : Inport  Port=10
  VarCompRatioPos : Inport  Port=11
  IntkVlvLift : Inport  Port=12
  VarIntkRunLen : Inport  Port=13
  IntkSwirlVlvPos : Inport  Port=14
  FuelFlw : Inport  Port=15
  FuelVolFlw : Inport  Port=16
  IntkPortFlow : Inport  Port=17
  NormAirChrg : Inport  Port=18
  ExhManGasTemp : Inport  Port=19
  Afr : Inport  Port=20
  TurboSpd : Inport  Port=21
  TurbPrsRatio : Inport  Port=22
  CompPrsRatio : Inport  Port=23
  TurbTempOut : Inport  Port=24
  CompTempOut : Inport  Port=25
  EgrPct : Inport  Port=26
  EgrMassFlwRate : Inport  Port=27
  EgrCoolerTempOut : Inport  Port=28
  IntercoolerTempOut : Inport  Port=29
  BSFC : Inport  Port=30
  TP HC : Inport  Port=31
  TP CO : Inport  Port=32
  TP NOx : Inport  Port=33
  TP CO2 : Inport  Port=34
  Iat : Inport  Port=35
  Ect : Inport  Port=36
  EgrVlvDeltaPrs : Inport  Port=37
  EgrVlvInTemp : Inport  Port=38
  Bus Creator1 : BusCreator  Inputs=37
  Terminator : Terminator
  EngFdbkOut : Outport  VectorParamsAs1DForOutWhenUnconnected=off
  wires:
  IntkSwirlVlvPos/1 -> Bus Creator1/14  "IntkSwirlVlvPos"
  VarIntkRunLen/1 -> Bus Creator1/13  "VarIntkRunLen"
  IntkVlvLift/1 -> Bus Creator1/12  "IntkVlvLift"
  VarCompRatioPos/1 -> Bus Creator1/11  "VarCompRatioPos"
  WgAreaPct/1 -> Bus Creator1/6  "WgAreaPct"
  TurboRackPos/1 -> Bus Creator1/9  "TurboRackPos"
  ThrPosPct/1 -> Bus Creator1/5  "ThrPosPct"
  EngTrq/1 -> Bus Creator1/1  "EngTrq"
  Mat/1 -> Bus Creator1/4  "Mat"
  Map/1 -> Bus Creator1/3  "Map"
  EngSpd/1 -> Bus Creator1/2  "EngSpd"
  Bus Creator1/1 -> EngFdbkOut/1  "EngFdbkOut"
  IntkCamPhase/1 -> Bus Creator1/7  "IntkCamPhase"
  ExhCamPhase/1 -> Bus Creator1/8  "ExhCamPhase"
  EgrVlvAreaPct/1 -> Bus Creator1/10  "EgrVlvAreaPct"
  FuelFlw/1 -> Bus Creator1/15  "FuelFlw"
  IntkPortFlow/1 -> Bus Creator1/16  "IntkPortFlow"
  NormAirChrg/1 -> Bus Creator1/17  "NormAirChrg"
  ExhManGasTemp/1 -> Bus Creator1/18  "ExhManGasTemp"
  Afr/1 -> Bus Creator1/19  "Afr"
  TurboSpd/1 -> Bus Creator1/20  "TurboSpd"
  TurbPrsRatio/1 -> Bus Creator1/21  "TurbPrsRatio"
  CompPrsRatio/1 -> Bus Creator1/22  "CompPrsRatio"
  TurbTempOut/1 -> Bus Creator1/23  "TurbTempOut"
  CompTempOut/1 -> Bus Creator1/24  "CompTempOut"
  IntercoolerTempOut/1 -> Bus Creator1/28  "IntercoolerTempOut"
  EgrPct/1 -> Bus Creator1/25  "EgrPct"
  EgrMassFlwRate/1 -> Bus Creator1/26  "EgrMassFlwRate"
  EgrCoolerTempOut/1 -> Bus Creator1/27  "EgrCoolerTempOut"
  BSFC/1 -> Bus Creator1/29  "BSFC"
  TP HC/1 -> Bus Creator1/30  "TP HC"
  TP CO/1 -> Bus Creator1/31  "TP CO"
  TP NOx/1 -> Bus Creator1/32  "TP NOx"
  TP CO2/1 -> Bus Creator1/33  "TP CO2"
  Ect/1 -> Bus Creator1/35  "Ect"
  EgrVlvDeltaPrs/1 -> Bus Creator1/36  "EgrVlvDeltaPrs"
  EgrVlvInTemp/1 -> Bus Creator1/37  "EgrVlvInTemp"
  Iat/1 -> Bus Creator1/34  "Iat"
  FuelVolFlw/1 -> Terminator/1  "FuelVolFlw"

== system SiDynoReferenceApplication/Performance Monitor/Waitbar/Function-Call Subsystem ==
  FracComplete : Inport
  function : TriggerPort  TriggerType=function-call  VariantControl=Variant
  Waitbar : MATLAB Function  TreatAsAtomicUnit=on
  wires:
  FracComplete/1 -> Waitbar/1(FracComplete)

== stateflow chart SiDynoReferenceApplication/Dynamometer Control/Steady State/Select Operating Point ==
  settings: executeAtInitialization=1
  state SetInitialPoint
    en:
    EngSpd = 0;
    TrqCmd = 0;
  state Startup
    en:
    EngSpd = EngSpdCmdPts(Index);
    TrqCmd = TrqCmdPts(Index);
    TotNumPoints = min(numel(EngSpdCmdPts), numel(TrqCmdPts));
  state LogData
    ex:
    LogDataTrigger = true;
  state WaitForSteadyState
    en:
    FracComplete = Index/TotNumPoints;
    LogDataTrigger = false;
  state SetNewValue
    en:
    Index = Index + 1;
    EngSpd = EngSpdCmdPts(Index);
    TrqCmd = TrqCmdPts(Index);
  state Stop
    en:
    FracComplete = 1;
    StopCmd = true;
  (default) -> SetInitialPoint : {
      | Index = 1;
      | StopCmd = false;
      | LogDataTrigger = false;
      | FracComplete = 0;
      | }
  SetInitialPoint -> Startup
  Startup -> WaitForSteadyState : after(5,sec)
  WaitForSteadyState -> LogData [order 2] : after(SteadyStateWaitLimit, sec)
  LogData -> (junction 73) : after(0.01, sec)
  (junction 73) -> SetNewValue [order 1] : [Index < numel(EngSpdCmdPts) || Index < numel(TrqCmdPts)]
  (junction 73) -> Stop [order 2]
  WaitForSteadyState -> LogData [order 1] : [SteadyStateFlag]
  SetNewValue -> WaitForSteadyState [order 1] : after(0.1,sec)[~SteadyStateFlag]
  SetNewValue -> WaitForSteadyState [order 2] : after(1.5,sec)
  data: SteadyStateFlag input; SteadyStateWaitLimit input; EngSpd output; EngSpdCmdPts input; TrqCmdPts input; TrqCmd output; Index local; LogDataTrigger output; StopCmd output; FracComplete output; TotNumPoints local

== matlab function SiDynoReferenceApplication/Performance Monitor/Waitbar/Function-Call Subsystem/Waitbar ==
  data: FracComplete input
function ShowWaitBar(FracComplete)
coder.extrinsic('waitbar', 'figure', 'findall'); 
h = findall(0, 'Type', 'figure', 'Tag', 'DynamometerWaitbarFig');
if ~isempty(h)
    waitbar(FracComplete, h(1));
end

== stateflow chart SiDynoReferenceApplication/Dynamometer Control/Calibrate Throttle and Wastegate/TPP and WAP Calibration Controller ==
  state CalibrationLoop [parallel]
    settings: executionOrder=2
    state TorqueControl [group]
      state WaitForSteadyState
        en:
        LogDataTrigger = false;
        during:
        TrqCmd = max(EngTrq, MinTrqCmd);
      state GotoMaxTrq
        en:
        LoadLoggedCtrlValues(2)
        during:
        TrqCmd = max(EngTrq, MinTrqCmd);
      state LogData
        en:
        LogDataTrigger = true;
      state CompleteTorquePoint
        en:
        EngTrq0 = EngTrq;
        FracComplete = min(max((EngSpdIndex - 1 + (TrqCmd - MinTrqCmd)/(MaxTrqCmd - MinTrqCmd))/numel(EngSpdBpts), FracComplete), 1);
        EngTrqOvershoot = false;
      state IncreaseTrqCmd
        en:
        LogDataTrigger = false;
        TrqCmd = TrqCmd + MinTrqStep;
      WaitForSteadyState -> (junction 1632) [order 2] : after(1, sec)
          | [(EngTrq - EngTrq0) > MaxTrqStep && SteadyStateFlag]
          | {DecreaseCtrlStep;
          | DecreaseCtrl;
          | EngTrqOvershoot = true;
          | MaxTrqReached = false;}
      (junction 1632) -> (junction 1639)
      WaitForSteadyState -> GotoMaxTrq [order 1] : [MaxTrqReached && ...
          | (EngTrq - EngTrq0) < MaxTrqStep &&...
          |  SteadyStateFlag]
      GotoMaxTrq -> (junction 1622) : after(1, sec)[SteadyStateFlag]
      (junction 1639) -> WaitForSteadyState
      (junction 1638) -> (junction 1639) : {IncreaseCtrl;}
      (junction 1624) -> WaitForSteadyState [order 2] : {LogCtrlValues(2);
          | IncreaseCtrl;}
      WaitForSteadyState -> CompleteTorquePoint [order 3] : [MinCtrlStepSizeReached]
          | {IncreaseCtrlStep;}
      WaitForSteadyState -> (junction 1640) [order 4] : after(1, sec)[SteadyStateFlag]
      (junction 1624) -> (junction 1622) [order 1] : [MaxTrqReached]
      (junction 1622) -> IncreaseTrqCmd [order 2]
      LogData -> (junction 1624) : after(0.01, sec)
      (junction 1637) -> (junction 1638) : {IncreaseCtrlStep;}
      (junction 1630) -> (junction 1637) [order 2]
      (junction 1623) -> (junction 1638) : {DecreaseCtrlStep;}
      (junction 1640) -> (junction 1630) [order 1] : [(EngTrq - EngTrq0) < MinTrqStep]
      (junction 1630) -> (junction 1623) [order 1] : [EngTrqOvershoot]
      (junction 1640) -> CompleteTorquePoint [order 2]
      CompleteTorquePoint -> LogData
      IncreaseTrqCmd -> CompleteTorquePoint : after(0.01, sec)
    state NewEngSpd [group]
      state AboveMinTrq
        during:
        TrqCmd = max(EngTrq, MinTrqCmd);
        MaxTrqReached = false;
      state BelowMinTrq
        during:
        MaxTrqReached = false;
        TrqCmd = max(EngTrq, MinTrqCmd);
      AboveMinTrq -> BelowMinTrq [order 1] : [EngTrq < MinTrqCmd - MinTrqStep...
          |  && ~MinCtrlStepSizeReached]
          | {DecreaseCtrlStep;
          | IncreaseCtrl;}
      BelowMinTrq -> AboveMinTrq [order 1] : [EngTrq > MinTrqCmd]
          | {DecreaseCtrlStep;
          | DecreaseCtrl;}
      (junction 1645) -> AboveMinTrq : {IncreaseCtrlStep;
          | DecreaseCtrl;}
      AboveMinTrq -> (junction 1670) [order 2] : after(1, sec)[SteadyStateFlag]
      (junction 1658) -> BelowMinTrq : {IncreaseCtrl;}
      BelowMinTrq -> (junction 1655) [order 2] : after(1, sec)[SteadyStateFlag]
      (junction 1670) -> (junction 1645) [order 2]
      (junction 1655) -> (junction 1658) [order 2]
      (junction 1670) -> (junction 1668) [order 1] : [MinCtrlStepSizeReached]
      (junction 1655) -> (junction 1659) [order 1] : [abs(EngTrq - MinTrqCmd) < MinTrqStep...
          | || MaxTrqReached]
      (junction 1668) -> (junction 1659)
    state Stop
      en:
      StopCmd = true;
    state GetMotoringTorque [group]
      state SetMotoringTorque
        en:
        TrqCmd = 0;
        CutOffFuel = 1;
      state LogMotoringData
        en:
        LogDataTrigger = true;
      state SetMinTrq
        en:
        TrqCmd = MinTrqCmd;
        CutOffFuel = 0;
        LogDataTrigger = false;
      SetMotoringTorque -> LogMotoringData : after(1, sec)[SteadyStateFlag]
      LogMotoringData -> SetMinTrq : after(0.01, sec)
    (default) -> (junction 1672) : {
        | EngSpdIndex = 0;
        | LoggedTPP = [0;0];
        | LoggedWAP = [0;0];
        | FracComplete = 0;
        | StartCtrl;
        | }
    (junction 1622) -> (junction 1672) [order 1] : [FracComplete >= ...
        | EngSpdIndex/numel(EngSpdBpts)]
    (junction 1672) -> BelowMinTrq [order 2] : {EngSpdIndex = EngSpdIndex + 1;
        | EngSpd = EngSpdBpts(EngSpdIndex);
        | LogDataTrigger = false;
        | ResetCtrl;
        | LoadLoggedCtrlValues(1); }
    (junction 1672) -> Stop [order 1] : [EngSpdIndex >= numel(EngSpdBpts)]
    (junction 1659) -> SetMotoringTorque : {LogCtrlValues(1);}
    SetMinTrq -> CompleteTorquePoint : after(1, sec)[SteadyStateFlag]
  state StartCtrl [function]
    (default) -> (junction 1687) : {
        | TPP = 5;
        | WAP = 100;
        | MaxCtrlStepSize = 5;
        | CtrlStepSize = 0.5;
        | LogCtrlValues(1)
        | LogCtrlValues(2)
        | }
  state DecreaseCtrl [function]
    (default) -> (junction 1442)
    (junction 1442) -> (junction 1439) [order 1] : [WAP < 100]
    (junction 1442) -> (junction 1443) [order 2] : {TPP = max(TPP - CtrlStepSize, 0);
        | WAP = 100;}
    (junction 1439) -> (junction 1444) : {WAP = min(WAP + CtrlStepSize, 100);
        | TPP = 100;}
    (junction 1444) -> (junction 1443)
    (junction 1443) -> (junction 1445)
  state DecreaseCtrlStep [function]
    (default) -> (junction 1491) : {CtrlStepSize = CtrlStepSize/2;
        | MinCtrlStepSize = 0.01;}
    (junction 1491) -> (junction 1490) [order 1] : [MinCtrlStepSize > CtrlStepSize]
    (junction 1491) -> (junction 1487) [order 2]
    (junction 1490) -> (junction 1489) : {CtrlStepSize = MinCtrlStepSize;
        | MinCtrlStepSizeReached = true;}
    (junction 1489) -> (junction 1487)
    (junction 1487) -> (junction 1452)
  state LogCtrlValues(Idx) [function]
    (default) -> (junction 1526) : {LoggedTPP(Idx) = TPP; LoggedWAP(Idx) = WAP;}
  state ResetCtrl [function]
    (default) -> (junction 1437) : {
        | CtrlStepSize = 0.5;
        | MinCtrlStepSizeReached = false;
        | }
  state IncreaseCtrl [function]
    (default) -> (junction 1455)
    (junction 1455) -> (junction 1456) [order 1] : [TPP >= 100]
    (junction 1455) -> (junction 1457) [order 2] : {TPP = min(TPP + CtrlStepSize, 100);
        | WAP = 100;}
    (junction 1456) -> (junction 1458) : {WAP = max(WAP - CtrlStepSize, 0);
        | TPP = 100;}
    (junction 1458) -> (junction 1457)
    (junction 1457) -> (junction 1459)
  state IncreaseCtrlStep [function]
    (default) -> (junction 1466) : {CtrlStepSize = min(2*CtrlStepSize, MaxCtrlStepSize);
        | MinCtrlStepSizeReached = false;}
  state LoadLoggedCtrlValues(Idx) [function]
    (default) -> (junction 1511) : {TPP = LoggedTPP(Idx); WAP = LoggedWAP(Idx);}
  state CheckTrqLimit [parallel]
    settings: executionOrder=1
    state TrqBelowMax
      en:
      MaxTrqReached = false;
    state TrqAboveMax
      en:
      MaxTrqReached = true;
    (default) -> TrqBelowMax
    TrqBelowMax -> TrqAboveMax : [TurboSpd > MaxTurboSpd || EngTrq > MaxTrqCmd ...
        | || WAP <= 0]
    TrqAboveMax -> TrqBelowMax : [~MaxTrqReached]
  data: Idx function_input; Idx function_input; SteadyStateFlag input; EngSpd output; TrqCmd output; EngSpdBpts input; MinTrqStep input; MaxTrqStep input; MinTrqCmd input; EngSpdIndex local; LogDataTrigger output; StopCmd output; FracComplete output; TPP output size=[1,1]; EngTrq0 local; WAP output size=[1,1]; MaxTrqCmd input; MaxTurboSpd input; EngTrq input; TurboSpd input; MaxTrqReached local; CtrlStepSize local; MaxCtrlStepSize local; MinCtrlStepSizeReached local; EngTrqOvershoot local; LoggedTPP local size=[2,1]; LoggedWAP local size=[2,1]; CutOffFuel output
